simulink model "LectureVersion_Stage05_ALL"  (R2021b)
settings: Solver=VariableStepAuto  StartTime=0.0  StopTime=24  RelTol=1e-3
model workspace: external: MAT-File params.mat (data not in the file)
undefined symbols (not defined in the file or in its folder): c_air, InitBias, M_heater_air, m_room_air, R_equivalent, T_heater, TARGET_TEMP, Troom_IC
settings Model: Creator=jim  LastModifiedBy=jim

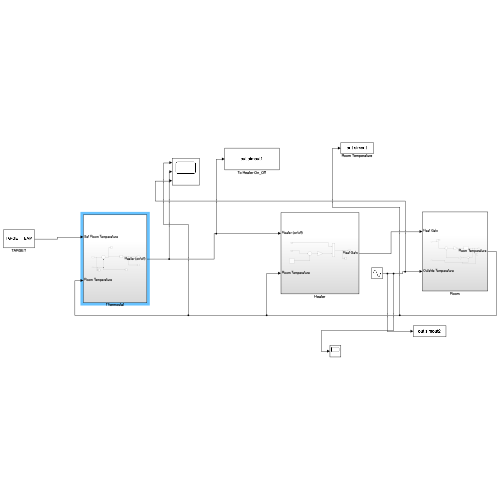
[thumbnail: Simulink's stored preview of the top-level diagram]
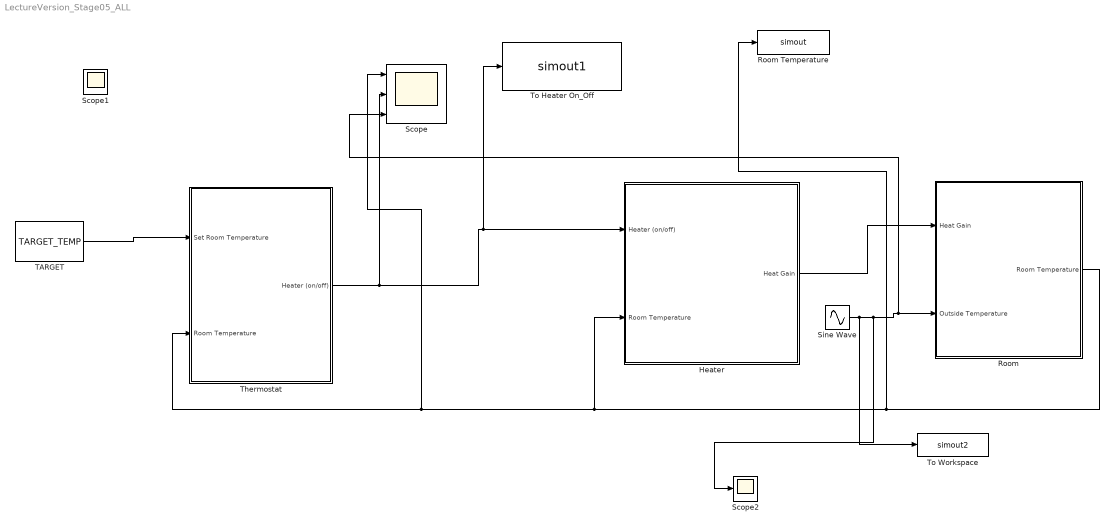
== system LectureVersion_Stage05_ALL ==
  Heater : Subsystem
  Room : Subsystem
  Room Temperature : ToWorkspace  VariableName=simout  SaveFormat=Timeseries  SampleTime=-1
  Scope : Scope  NumInputPorts=3
  Scope2 : Scope
  Sine Wave : Sin  Amplitude=5  Bias=InitBias  Frequency=2*pi/24  Phase=180  SampleTime=0
  TARGET : Constant  Value=TARGET_TEMP
  Thermostat : Subsystem
  To Heater On_Off : ToWorkspace  VariableName=simout1  SaveFormat=Timeseries  SampleTime=-1
  To Workspace : ToWorkspace  VariableName=simout2  SaveFormat=Timeseries  SampleTime=-1
  Scope1 : Scope
  wires:
  TARGET/1 -> Thermostat/1(Set Room Temperature)
  Thermostat/1(Heater (on/off)) -> Scope/2, Heater/1(Heater (on/off)), To Heater On_Off/1
  Room/1(Room Temperature) -> Room Temperature/1, Heater/2(Room Temperature), Scope/1, Thermostat/2(Room Temperature)
  Heater/1(Heat Gain) -> Room/1(Heat Gain)
  Sine Wave/1 -> To Workspace/1, Scope2/1, Scope/3, Room/2(Outside Temperature)

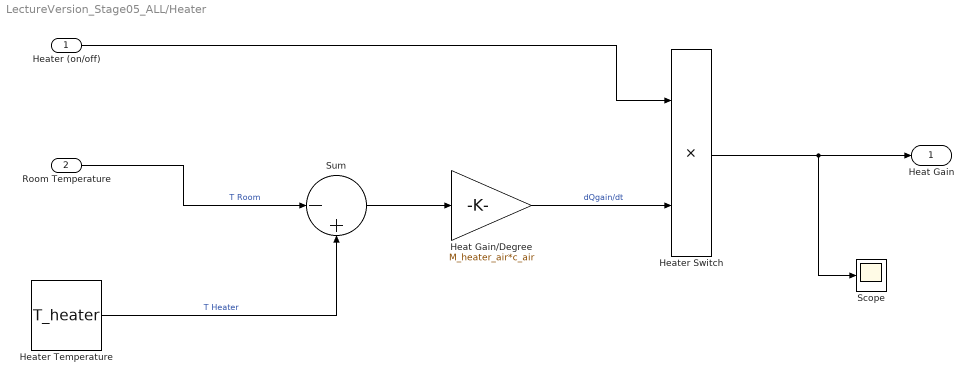
== system LectureVersion_Stage05_ALL/Heater ==
  Heater (on/off) : Inport
  Room Temperature : Inport  Port=2
  Heat Gain/Degree : Gain  Gain=M_heater_air*c_air
  Heater Switch : Product
  Heater Temperature : Constant  Value=T_heater
  Scope : Scope
  Sum : Sum  Inputs=|-+
  Heat Gain : Outport
  wires:
  Sum/1 -> Heat Gain/Degree/1
  Room Temperature/1 -> Sum/1  "T Room"
  Heater Temperature/1 -> Sum/2  "T Heater"
  Heater (on/off)/1 -> Heater Switch/1
  Heater Switch/1 -> Scope/1, Heat Gain/1
  Heat Gain/Degree/1 -> Heater Switch/2  "dQgain/dt"

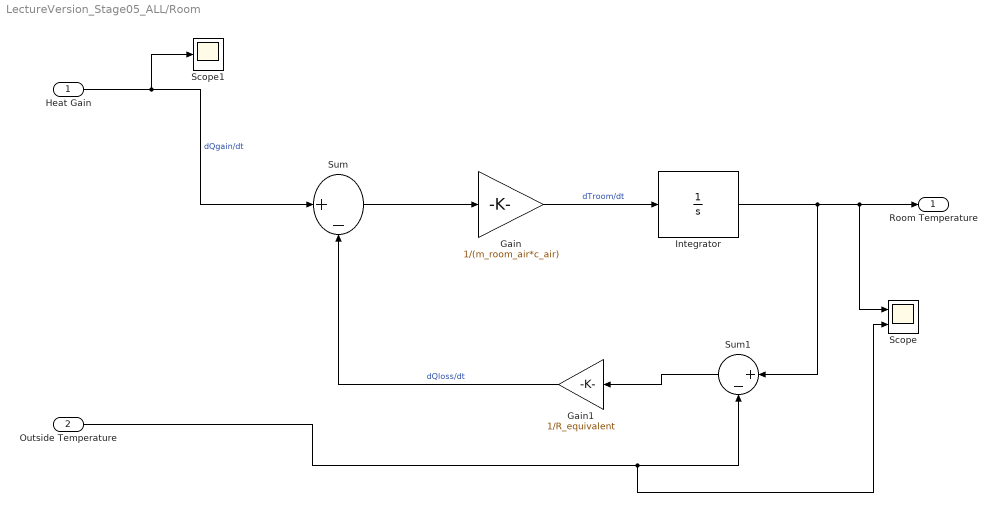
== system LectureVersion_Stage05_ALL/Room ==
  Heat Gain : Inport
  Outside Temperature : Inport  Port=2
  Gain : Gain  Gain=1/(m_room_air*c_air)
  Gain1 : Gain  Gain=1/R_equivalent
  Integrator : Integrator  InitialCondition=Troom_IC
  Scope : Scope  NumInputPorts=2
  Scope1 : Scope
  Sum : Sum  Inputs=|+-
  Sum1 : Sum  Inputs=|+-
  Room Temperature : Outport
  wires:
  Heat Gain/1 -> Scope1/1, Sum/1  "dQgain/dt"
  Sum/1 -> Gain/1
  Gain/1 -> Integrator/1  "dTroom/dt"
  Gain1/1 -> Sum/2  "dQloss/dt"
  Integrator/1 -> Sum1/1, Scope/1, Room Temperature/1
  Outside Temperature/1 -> Scope/2, Sum1/2
  Sum1/1 -> Gain1/1

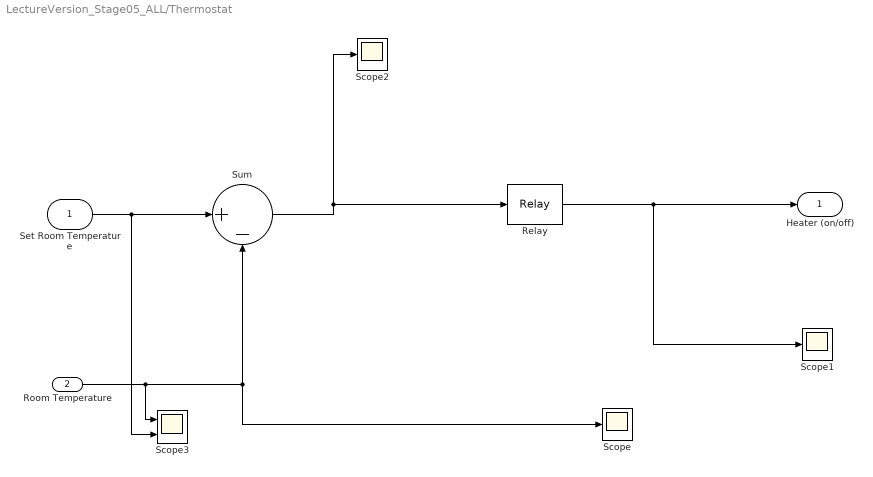
== system LectureVersion_Stage05_ALL/Thermostat ==
  Set Room Temperature : Inport
  Room Temperature : Inport  Port=2
  Relay : Relay  OnSwitchValue=2  OffSwitchValue=-2
  Scope : Scope
  Scope1 : Scope
  Scope2 : Scope
  Scope3 : Scope  NumInputPorts=2
  Sum : Sum  Inputs=|+-
  Heater (on/off) : Outport
  wires:
  Set Room Temperature/1 -> Sum/1, Scope3/2
  Room Temperature/1 -> Scope3/1, Sum/2, Scope/1
  Sum/1 -> Relay/1, Scope2/1
  Relay/1 -> Scope1/1, Heater (on/off)/1
